simulink model "BallBeam"  (R2024a)
settings: Solver=VariableStepAuto  StartTime=0.0  StopTime=1  MaxStep=1e-3  RelTol=1e-3
settings Model: Creator=perruquetti  LastModifiedBy=perruquetti

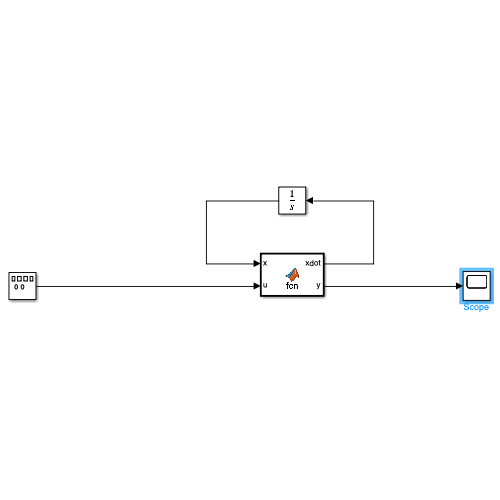
[thumbnail: Simulink's stored preview of the top-level diagram]
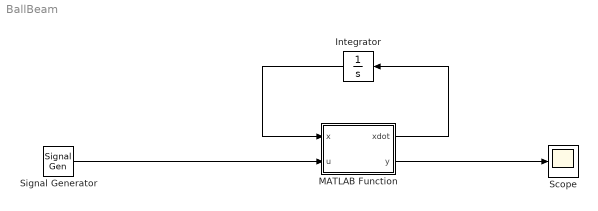
== system BallBeam ==
  Integrator : Integrator  InitialCondition="[0.012;  0; 0.84;0]"
  MATLAB Function : MATLAB Function  TreatAsAtomicUnit=on
  Scope : Scope
  Signal Generator : SignalGenerator  Amplitude=10  Frequency=100  Units=rad/sec
  wires:
  MATLAB Function/1(xdot) -> Integrator/1
  Integrator/1 -> MATLAB Function/1(x)
  MATLAB Function/2(y) -> Scope/1
  Signal Generator/1 -> MATLAB Function/2(u)

== matlab function BallBeam/MATLAB Function ==
  data: x input; xdot output; u input; y output
function [xdot,y] = fcn(x,u)
%\dot x_1&=& x_2,\\
%\dot x_2&=& -g\sin (x_3 )+x_1x_3^{2}\\
%\dot x_3&=& x_4,\\
%\dot x_4&=& \frac{1}{(mx_1^{2}+J)} \left( u-2m x_1x_2x_4-mgx_1\cos (x_3 )\right),
% constants
    m = 0.1; 
    J = 0.1;
    g = 9.81;
% nonlinear set of equations
    xdot = [x(2);
        -g*sin(x(3))+x(1)*x(3)*x(3);
        x(4);
        (u(1)-2*m*x(1)*x(2)*x(4)-m*g*x(1)*cos(x(3)))/(m*x(1)*x(1)+J)];
    y = x';
